simulink model "dm_modified"  (R2018a)
settings: Solver=VariableStepAuto  StartTime=0.0  StopTime=2  RelTol=1e-3
libraries: dspquant2 x2, dsparch4 x1
settings Model: Creator=hp  LastModifiedBy=hp

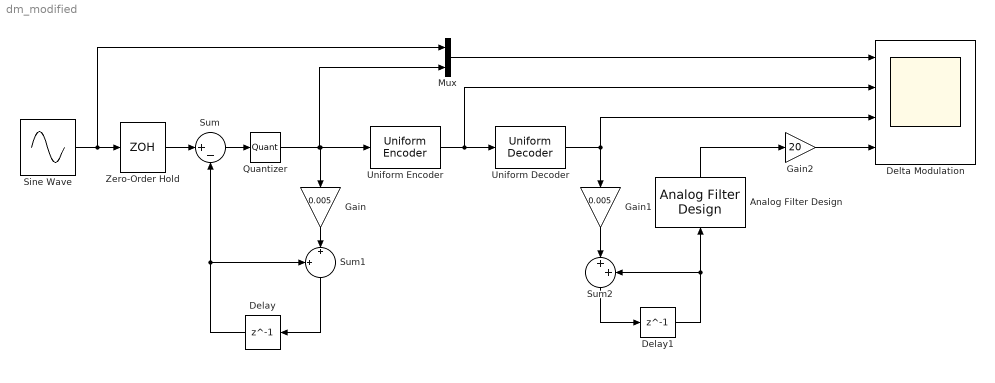
== system dm_modified ==
  " Delay" : Delay  DelayLength=1
  " Sum1" : Sum  Inputs=+|+||
  " Sum2" : Sum  Inputs=|++
  "            Sum" : Sum  Inputs=|+-
  Analog Filter Design : dsparch4/Analog Filter Design  method=Butterworth  filttype=Lowpass  N=8  Wlo=2*pi*12  Whi=80  Rp=2  Rs=40
  Delay1 : Delay  DelayLength=1
  Delta Modulation : Scope  NumInputPorts=4
  Gain : Gain  Gain=0.005
  Gain1 : Gain  Gain=0.005
  Gain2 : Gain  Gain=20
  Mux : Mux  Inputs=2
  Quantizer : Quantizer
  Sine Wave : Sin  Frequency=2*pi*10  SampleTime=0
  Uniform Decoder : dspquant2/Uniform Decoder  peak=2  bits=8  overflowMode=Saturate  otype=Double
      settings: SourceProductName=DSP System Toolbox  SourceProductBaseCode=DS
  Uniform Encoder : dspquant2/Uniform Encoder  peak=2  bits=8  otype=Signed integer
      settings: SourceProductName=DSP System Toolbox
  Zero-Order Hold : ZeroOrderHold  SampleTime=1/100
  wires:
  " Sum1"/1 -> " Delay"/1
  Uniform Decoder/1 -> Delta Modulation/3, Gain1/1
  " Delay"/1 -> " Sum1"/1, "            Sum"/2
  Mux/1 -> Delta Modulation/1
  Analog Filter Design/1 -> Gain2/1
  Gain2/1 -> Delta Modulation/4
  Uniform Encoder/1 -> Delta Modulation/2, Uniform Decoder/1
  " Sum2"/1 -> Delay1/1
  Sine Wave/1 -> Mux/1, Zero-Order Hold/1
  Quantizer/1 -> Uniform Encoder/1, Gain/1, Mux/2
  Gain1/1 -> " Sum2"/1
  "            Sum"/1 -> Quantizer/1
  Delay1/1 -> " Sum2"/2, Analog Filter Design/1
  Gain/1 -> " Sum1"/2
  Zero-Order Hold/1 -> "            Sum"/1
